simulink library "SensAdapt_lib"  (R2013a)
settings: Solver=ode45  StartTime=0.0  StopTime=10.0  RelTol=1e-3
libraries: simulink x1
settings Model: Creator=User  LastModifiedBy=User

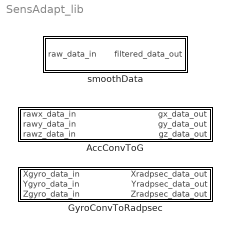
== system SensAdapt_lib ==
  AccConvToG : Subsystem  TreatAsAtomicUnit=on
      settings: RTWSystemCode=Nonreusable function  RTWFcnNameOpts=Use subsystem name
  GyroConvToRadpsec : Subsystem  TreatAsAtomicUnit=on
      settings: RTWSystemCode=Nonreusable function  RTWFcnNameOpts=Use subsystem name
  smoothData : Subsystem  TreatAsAtomicUnit=on
      settings: RTWSystemCode=Nonreusable function  RTWFcnNameOpts=Use subsystem name

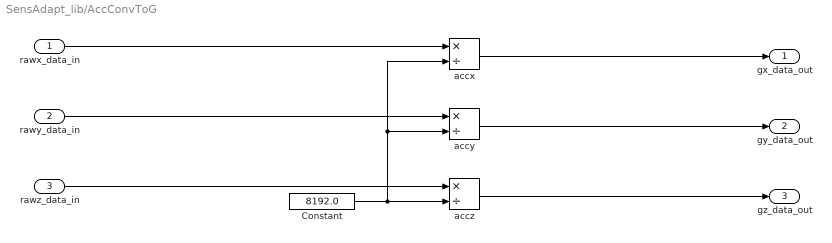
== system SensAdapt_lib/AccConvToG ==
  rawx_data_in : Inport
  rawy_data_in : Inport  Port=2
  rawz_data_in : Inport  Port=3
  Constant : Constant  Value=8192.0
  accx : Product  Inputs=*/
  accy : Product  Inputs=*/
  accz : Product  Inputs=*/
  gx_data_out : Outport  OutDataTypeStr=double
  gy_data_out : Outport  Port=2  OutDataTypeStr=double
  gz_data_out : Outport  Port=3  OutDataTypeStr=double
  wires:
  Constant/1 -> accx/2, accy/2, accz/2
  rawx_data_in/1 -> accx/1
  rawy_data_in/1 -> accy/1
  rawz_data_in/1 -> accz/1
  accy/1 -> gy_data_out/1
  accz/1 -> gz_data_out/1
  accx/1 -> gx_data_out/1

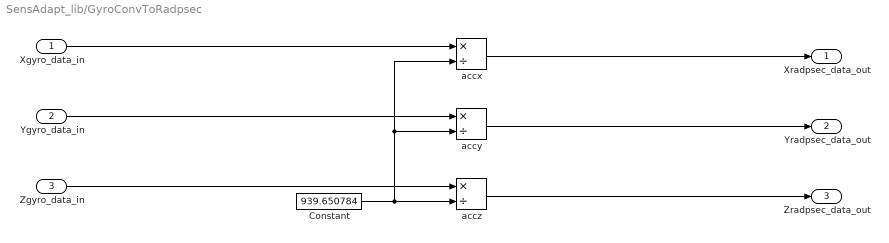
== system SensAdapt_lib/GyroConvToRadpsec ==
  Xgyro_data_in : Inport
  Ygyro_data_in : Inport  Port=2
  Zgyro_data_in : Inport  Port=3
  Constant : Constant  Value=939.650784
  accx : Product  Inputs=*/
  accy : Product  Inputs=*/
  accz : Product  Inputs=*/
  Xradpsec_data_out : Outport  OutDataTypeStr=double
  Yradpsec_data_out : Outport  Port=2  OutDataTypeStr=double
  Zradpsec_data_out : Outport  Port=3  OutDataTypeStr=double
  wires:
  accx/1 -> Xradpsec_data_out/1
  accz/1 -> Zradpsec_data_out/1
  accy/1 -> Yradpsec_data_out/1
  Zgyro_data_in/1 -> accz/1
  Ygyro_data_in/1 -> accy/1
  Xgyro_data_in/1 -> accx/1
  Constant/1 -> accz/2, accy/2, accx/2

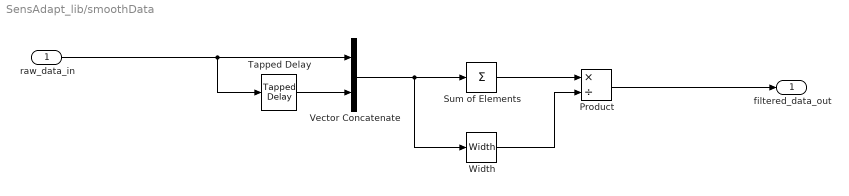
== system SensAdapt_lib/smoothData ==
  raw_data_in : Inport
  Product : Product  Inputs=*/  OutDataTypeStr=double
  Sum of Elements : Sum  Inputs=+  AccumDataTypeStr=double  OutDataTypeStr=double
  Tapped Delay : simulink/Discrete/Tapped Delay  vinit=9  samptime=-1  NumDelays=9  DelayOrder=Oldest  includeCurrent=off
  Vector Concatenate : Concatenate
  Width : Width  DataType=uint16
  filtered_data_out : Outport  OutDataTypeStr=double
  wires:
  raw_data_in/1 -> Vector Concatenate/1, Tapped Delay/1
  Product/1 -> filtered_data_out/1
  Width/1 -> Product/2
  Sum of Elements/1 -> Product/1
  Vector Concatenate/1 -> Sum of Elements/1, Width/1
  Tapped Delay/1 -> Vector Concatenate/2
